simulink model "detumbling1"  (R2022b)
settings: Solver=ode5  StartTime=startTime  StopTime=stopTime  FixedStep=stepsize  RelTol=1e-3
undefined symbols (not defined in the file): a, A_BN0, ARW, c, detumblingkb, detumblingkp, e, EHAccuracy, EHSampleRate, first_detumbling_time_1RW, G, GyroSampleRate, H, h_RW_max, i, inertia1, inertia2, inertia3, Inertia_matrix, Inverse_inertia, Ld, Lw, m, maxdipole, MB, MMnoise, MMSampleRate, mu, n, R_e, rho_d_MB, rho_d_SP, rho_s_MB, rho_s_SP, RRW, SP, theta0, torque_RW_max, w0, wheel_axis
libraries: matrix_library x11, vrlib x10, simulink_extras x4
(part 2 of 3)

== system detumbling1/External Torques/Solar radiation/Torque arm SP ==
  SP : Inport
  A_vect_SP : Inport  Port=2
  S_B : Inport  Port=3
  pointer_SP : Inport  Port=4
  r_SP1 : Inport  Port=5
  r_SP2 : Inport  Port=6
  Add : Sum
  Add1 : Sum
  Reshape : Reshape  OutputDimensionality=Customize  OutputDimensions=[2,3]
  Vector Concatenate : Concatenate
  creazione raggi vettore tra CM SP e centro facce illuminate della faccia che ha come normale l'asse j : Subsystem
  distance : Outport
  wires:
  Reshape/1 -> distance/1
  SP/1 -> [SP]
  A_vect_SP/1 -> [A_vect_SP]
  S_B/1 -> [S_B]
  pointer_SP/1 -> [pointer_SP]
  r_SP1/1 -> [r_SP1]
  r_SP2/1 -> [r_SP2]
  [S_B] -> creazione raggi vettore tra CM SP e centro facce illuminate della faccia che ha come normale l'asse j/1(S_B)
  [SP] -> creazione raggi vettore tra CM SP e centro facce illuminate della faccia che ha come normale l'asse j/2(SP)
  [A_vect_SP] -> creazione raggi vettore tra CM SP e centro facce illuminate della faccia che ha come normale l'asse j/3(A_vect)
  [pointer_SP] -> creazione raggi vettore tra CM SP e centro facce illuminate della faccia che ha come normale l'asse j/4(pointer)
  creazione raggi vettore tra CM SP e centro facce illuminate della faccia che ha come normale l'asse j/1(distance) -> [distance]
  Vector Concatenate/1 -> Reshape/1
  Add/1 -> Vector Concatenate/1
  [distance] -> Add/1
  [r_SP1] -> Add/2
  [r_SP2] -> Add1/2
  [distance] -> Add1/1
  Add1/1 -> Vector Concatenate/2

== system detumbling1/Sensors/Earth Horizon Sensor/A_eps ==
  Constant : Constant
  Display : Display
  Gain : Gain  Gain=[1; -1; 1]
  Gain1 : Gain  Gain=[1; 1; -1]
  Gain2 : Gain  Gain=[-1; 1; 1]
  Matrix Concatenate : Concatenate  NumInputs=3  Mode=Multidimensional array  ConcatenateDimension=2
  Random Number : RandomNumber  Variance=deg2rad(EHAccuracy)^2  Seed=5  SampleTime=1/EHSampleRate
  Random Number1 : RandomNumber  Variance=deg2rad(EHAccuracy)^2  Seed=6  SampleTime=1/EHSampleRate
  Random Number2 : RandomNumber  Variance=deg2rad(EHAccuracy)^2  Seed=7  SampleTime=1/EHSampleRate
  Selector : Selector  InputPortWidth=4  IndexOptions=Index vector (dialog)  Indices=[1 4 3]  OutputSizes=1
  Selector1 : Selector  InputPortWidth=4  IndexOptions=Index vector (dialog)  Indices=[4 1 2 ]  OutputSizes=1
  Selector2 : Selector  InputPortWidth=4  IndexOptions=Index vector (dialog)  Indices=[3 2 1]  OutputSizes=1
  Vector Concatenate : Concatenate  NumInputs=4
  A_epsHS : Outport
  wires:
  Selector/1 -> Gain/1
  Matrix Concatenate/1 -> A_epsHS/1, Display/1
  Random Number/1 -> Vector Concatenate/2
  Vector Concatenate/1 -> Selector2/1, Selector/1, Selector1/1
  Selector1/1 -> Gain1/1
  Gain/1 -> Matrix Concatenate/1
  Selector2/1 -> Gain2/1
  Gain2/1 -> Matrix Concatenate/3
  Gain1/1 -> Matrix Concatenate/2
  Constant/1 -> Vector Concatenate/1
  Random Number2/1 -> Vector Concatenate/4
  Random Number1/1 -> Vector Concatenate/3

== system detumbling1/Sensors/Magnetometer/Subsystem ==
  Constant : Constant
  Display : Display
  Gain : Gain  Gain=[1; -1; 1]
  Gain1 : Gain  Gain=[1; 1; -1]
  Gain2 : Gain  Gain=[-1; 1; 1]
  Matrix Concatenate : Concatenate  NumInputs=3  Mode=Multidimensional array  ConcatenateDimension=2
  Random Number : RandomNumber  Variance=deg2rad(0.1)^2  Seed=5  SampleTime=1/MMSampleRate
  Random Number1 : RandomNumber  Variance=deg2rad(0.1)^2  Seed=6  SampleTime=1/MMSampleRate
  Random Number2 : RandomNumber  Variance=deg2rad(0.1)^2  Seed=7  SampleTime=1/MMSampleRate
  Selector : Selector  InputPortWidth=4  IndexOptions=Index vector (dialog)  Indices=[1 4 3]  OutputSizes=1
  Selector1 : Selector  InputPortWidth=4  IndexOptions=Index vector (dialog)  Indices=[4 1 2]  OutputSizes=1
  Selector2 : Selector  InputPortWidth=4  IndexOptions=Index vector (dialog)  Indices=[3 2 1]  OutputSizes=1
  Vector Concatenate : Concatenate  NumInputs=4
  A_epsMM : Outport
  wires:
  Selector2/1 -> Gain2/1
  Selector/1 -> Gain/1
  Gain/1 -> Matrix Concatenate/1
  Random Number/1 -> Vector Concatenate/2
  Matrix Concatenate/1 -> Display/1, A_epsMM/1
  Selector1/1 -> Gain1/1
  Vector Concatenate/1 -> Selector2/1, Selector/1, Selector1/1
  Gain2/1 -> Matrix Concatenate/3
  Constant/1 -> Vector Concatenate/1
  Gain1/1 -> Matrix Concatenate/2
  Random Number2/1 -> Vector Concatenate/4
  Random Number1/1 -> Vector Concatenate/3

== system detumbling1/External Torques/Solar radiation/Force MB/Subsystem ==
  S_B : Inport
  N_MB : Inport  Port=2
  Constant3 : Constant  Value=[1, 1, 1]
  Matrix Multiply5 : Product  Multiplication=Matrix(*)
  Product10 : Product
  Reshape11 : Reshape  OutputDimensionality=Row vector (2-D)
  Reshape12 : Reshape  OutputDimensionality=Column vector (2-D)
  Sum of Elements : Sum  Inputs=+  CollapseMode=Specified dimension  CollapseDim=2
  Out1 : Outport
  wires:
  Matrix Multiply5/1 -> Product10/1
  Reshape12/1 -> Matrix Multiply5/1
  S_B/1 -> Reshape12/1
  Product10/1 -> Sum of Elements/1
  N_MB/1 -> Product10/2
  Sum of Elements/1 -> Out1/1
  Constant3/1 -> Reshape11/1
  Reshape11/1 -> Matrix Multiply5/2

== system detumbling1/External Torques/Solar radiation/Inertia matrix/r_SP ==
  b_SP : Inport
  a_MB : Inport  Port=2
  Constant : Constant  Value=[1 0 0]
  Gain : Gain  Gain=1/2
  Gain1 : Gain  Gain=1/2
  Gain2 : Gain  Gain=-1
  Product : Product
  Reshape : Reshape  OutputDimensionality=Column vector (2-D)
  Sum : Sum
  r_SP1 : Outport
  r_SP2 : Outport  Port=2
  wires:
  Constant/1 -> Reshape/1
  a_MB/1 -> Gain/1
  b_SP/1 -> Gain1/1
  Gain1/1 -> Sum/1
  Gain/1 -> Sum/2
  Reshape/1 -> Product/1
  Sum/1 -> Product/2
  Gain2/1 -> r_SP2/1
  Product/1 -> r_SP1/1, Gain2/1

== system detumbling1/External Torques/Solar radiation/S_B dot N_MB/If Action Subsystem ==
  NMB : Inport
  Action Port : ActionPort  ActionPortLabel=if(u1 > 0)
  Constant : Constant
  Selector : Selector  NumberOfDimensions=2  InputPortWidth=3  IndexOptions=Index vector (dialog),Index vector (dialog)  Indices=1,[1 2 3]  OutputSizes=1,1
  x : Outport
  pointer : Outport  Port=2
  wires:
  NMB/1 -> Selector/1
  Selector/1 -> x/1
  Constant/1 -> pointer/1

== system detumbling1/External Torques/Solar radiation/S_B dot N_MB/If Action Subsystem1 ==
  NMB : Inport
  Action Port : ActionPort  ActionPortLabel=if(u1 > 0)
  Constant : Constant
  Selector : Selector  NumberOfDimensions=2  InputPortWidth=3  IndexOptions=Index vector (dialog),Index vector (dialog)  Indices=2,[1 2 3]  OutputSizes=1,1
  y : Outport
  pointer : Outport  Port=2
  wires:
  Selector/1 -> y/1
  NMB/1 -> Selector/1
  Constant/1 -> pointer/1

== system detumbling1/External Torques/Solar radiation/S_B dot N_MB/If Action Subsystem2 ==
  NMB : Inport
  Action Port : ActionPort  ActionPortLabel=if(u1 > 0)
  Constant : Constant
  Selector : Selector  NumberOfDimensions=2  InputPortWidth=3  IndexOptions=Index vector (dialog),Index vector (dialog)  Indices=3,[1 2 3]  OutputSizes=1,1
  z : Outport
  pointer : Outport  Port=2
  wires:
  NMB/1 -> Selector/1
  Selector/1 -> z/1
  Constant/1 -> pointer/1

== system detumbling1/External Torques/Solar radiation/S_B dot N_MB/If Action Subsystem3 ==
  NMB : Inport
  Action Port : ActionPort  ActionPortLabel=else
  Constant : Constant  Value=-1
  Selector : Selector  NumberOfDimensions=2  InputPortWidth=3  IndexOptions=Index vector (dialog),Index vector (dialog)  Indices=4,[1 2 3]  OutputSizes=1,1
  -x : Outport
  pointer : Outport  Port=2
  wires:
  Selector/1 -> -x/1
  NMB/1 -> Selector/1
  Constant/1 -> pointer/1

== system detumbling1/External Torques/Solar radiation/S_B dot N_MB/If Action Subsystem4 ==
  NMB : Inport
  Action Port : ActionPort  ActionPortLabel=else
  Constant : Constant  Value=-1
  Selector : Selector  NumberOfDimensions=2  InputPortWidth=3  IndexOptions=Index vector (dialog),Index vector (dialog)  Indices=5,[1 2 3]  OutputSizes=1,1
  -y : Outport
  pointer : Outport  Port=2
  wires:
  NMB/1 -> Selector/1
  Selector/1 -> -y/1
  Constant/1 -> pointer/1

== system detumbling1/External Torques/Solar radiation/S_B dot N_MB/If Action Subsystem5 ==
  NMB : Inport
  Action Port : ActionPort  ActionPortLabel=else
  Constant : Constant  Value=-1
  Selector : Selector  NumberOfDimensions=2  InputPortWidth=3  IndexOptions=Index vector (dialog),Index vector (dialog)  Indices=6,[1 2 3]  OutputSizes=1,1
  -z : Outport
  pointer : Outport  Port=2
  wires:
  Selector/1 -> -z/1
  NMB/1 -> Selector/1
  Constant/1 -> pointer/1

== system detumbling1/External Torques/Solar radiation/S_B dot N_SP/If Action Subsystem ==
  N_SP : Inport
  Action Port : ActionPort  ActionPortLabel=if(u1 > 0)
  Constant : Constant
  Selector : Selector  NumberOfDimensions=2  InputPortWidth=3  IndexOptions=Index vector (dialog),Index vector (dialog)  Indices=1,[1 2 3]  OutputSizes=1,1
  true_NSP : Outport
  pointer : Outport  Port=2
  wires:
  N_SP/1 -> Selector/1
  Constant/1 -> pointer/1
  Selector/1 -> true_NSP/1

== system detumbling1/External Torques/Solar radiation/S_B dot N_SP/If Action Subsystem1 ==
  N_SP : Inport
  Action Port : ActionPort  ActionPortLabel=if(u1 > 0)
  Constant : Constant  Value=-1
  Selector : Selector  NumberOfDimensions=2  InputPortWidth=3  IndexOptions=Index vector (dialog),Index vector (dialog)  Indices=2,[1 2 3]  OutputSizes=1,1
  true_NSP : Outport
  pointer : Outport  Port=2
  wires:
  Selector/1 -> true_NSP/1
  Constant/1 -> pointer/1
  N_SP/1 -> Selector/1

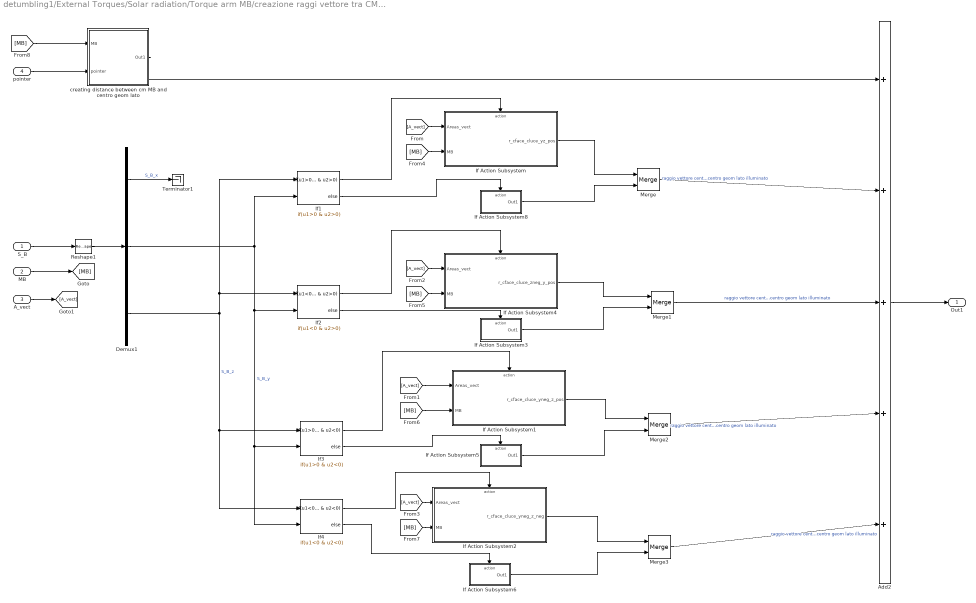
== system detumbling1/External Torques/Solar radiation/Torque arm MB/creazione raggi vettore tra CM MB e centro facce illuminate della faccia che ha come normale l'asse i ==
  S_B : Inport
  MB : Inport  Port=2
  A_vect : Inport  Port=3
  pointer : Inport  Port=4
  Add2 : Sum  Inputs=+|+|+|+|+
  Demux1 : Demux  Outputs=3
  If Action Subsystem : Subsystem  TreatAsAtomicUnit=on
  If Action Subsystem1 : Subsystem  TreatAsAtomicUnit=on
  If Action Subsystem2 : Subsystem  TreatAsAtomicUnit=on
  If Action Subsystem3 : Subsystem  TreatAsAtomicUnit=on
  If Action Subsystem4 : Subsystem  TreatAsAtomicUnit=on
  If Action Subsystem5 : Subsystem  TreatAsAtomicUnit=on
  If Action Subsystem6 : Subsystem  TreatAsAtomicUnit=on
  If Action Subsystem8 : Subsystem  TreatAsAtomicUnit=on
  If1 : If  NumInputs=2  IfExpression=u1>0 & u2>0
  If2 : If  NumInputs=2  IfExpression=u1<0 & u2>0
  If3 : If  NumInputs=2  IfExpression=u1>0 & u2<0
  If4 : If  NumInputs=2  IfExpression=u1<0 & u2<0
  Merge{,1..3} (4 alike) : Merge
  Reshape1 : Reshape  OutputDimensionality=Column vector (2-D)
  Terminator1 : Terminator
  creating distance between cm MB and centro geom lato : Subsystem
  Out1 : Outport
  wires:
  [A_vect] -> If Action Subsystem2/1(Areas_vect)
  [A_vect] -> If Action Subsystem1/1(Areas_vect)
  [A_vect] -> If Action Subsystem4/1(Areas_vect)
  Add2/1 -> Out1/1
  Merge3/1 -> Add2/5  "raggio vettore centro geom lato- centro geom lato illuminato"
  If4/1 -> If Action Subsystem2/Action
  If Action Subsystem2/1(r_cface_cluce_yneg_z_neg) -> Merge3/1
  If3/1 -> If Action Subsystem1/Action
  [A_vect] -> If Action Subsystem/1(Areas_vect)
  Merge1/1 -> Add2/3  "raggio vettore centro geom lato- centro geom lato illuminato"
  If Action Subsystem4/1(r_cface_cluce_zneg_y_pos) -> Merge1/1
  Merge/1 -> Add2/2  "raggio vettore centro geom lato- centro geom lato illuminato"
  If Action Subsystem/1(r_cface_cluce_yz_pos) -> Merge/1
  If1/2 -> If Action Subsystem8/Action
  S_B/1 -> Reshape1/1
  Reshape1/1 -> Demux1/1
  Demux1/2 -> If2/2, If3/2, If4/2, If1/2  "S_B_y"
  If2/1 -> If Action Subsystem4/Action
  If1/1 -> If Action Subsystem/Action
  Demux1/3 -> If4/1, If3/1, If2/1, If1/1  "S_B_z"
  creating distance between cm MB and centro geom lato/1(Out1) -> Add2/1
  Demux1/1 -> Terminator1/1  "S_B_x"
  MB/1 -> [MB]
  [MB] -> If Action Subsystem/2(MB)
  [MB] -> If Action Subsystem4/2(MB)
  [MB] -> If Action Subsystem1/2(MB)
  [MB] -> If Action Subsystem2/2(MB)
  If Action Subsystem8/1(Out1) -> Merge/2
  If2/2 -> If Action Subsystem3/Action
  If3/2 -> If Action Subsystem5/Action
  If4/2 -> If Action Subsystem6/Action
  If Action Subsystem3/1(Out1) -> Merge1/2
  If Action Subsystem1/1(r_cface_cluce_yneg_z_pos) -> Merge2/1
  If Action Subsystem5/1(Out1) -> Merge2/2
  Merge2/1 -> Add2/4  "raggio vettore centro geom lato- centro geom lato illuminato"
  If Action Subsystem6/1(Out1) -> Merge3/2
  [MB] -> creating distance between cm MB and centro geom lato/1(MB)
  A_vect/1 -> [A_vect]
  pointer/1 -> creating distance between cm MB and centro geom lato/2(pointer)

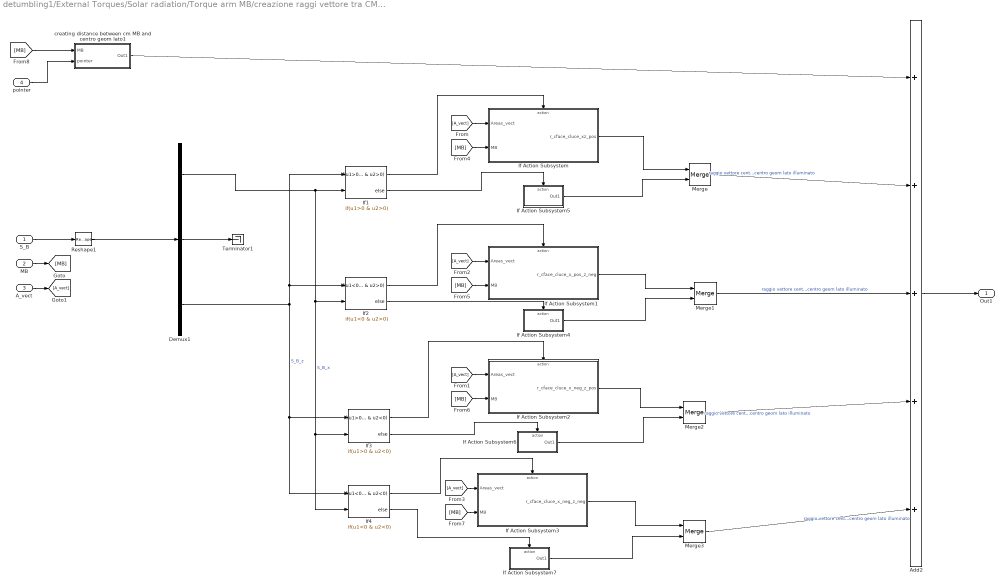
== system detumbling1/External Torques/Solar radiation/Torque arm MB/creazione raggi vettore tra CM MB e centro facce illuminate della faccia che ha come normale l'asse j ==
  S_B : Inport
  MB : Inport  Port=2
  A_vect : Inport  Port=3
  pointer : Inport  Port=4
  Add2 : Sum  Inputs=+|+|+|+|+
  Demux1 : Demux  Outputs=3
  If Action Subsystem : Subsystem  TreatAsAtomicUnit=on
  If Action Subsystem1 : Subsystem  TreatAsAtomicUnit=on
  If Action Subsystem2 : Subsystem  TreatAsAtomicUnit=on
  If Action Subsystem3 : Subsystem  TreatAsAtomicUnit=on
  If Action Subsystem4 : Subsystem  TreatAsAtomicUnit=on
  If Action Subsystem5 : Subsystem  TreatAsAtomicUnit=on
  If Action Subsystem6 : Subsystem  TreatAsAtomicUnit=on
  If Action Subsystem7 : Subsystem  TreatAsAtomicUnit=on
  If1 : If  NumInputs=2  IfExpression=u1>0 & u2>0
  If2 : If  NumInputs=2  IfExpression=u1<0 & u2>0
  If3 : If  NumInputs=2  IfExpression=u1>0 & u2<0
  If4 : If  NumInputs=2  IfExpression=u1<0 & u2<0
  Merge{,1..3} (4 alike) : Merge
  Reshape1 : Reshape  OutputDimensionality=Column vector (2-D)
  Terminator1 : Terminator
  creating distance between cm MB and centro geom lato1 : Subsystem
  Out1 : Outport
  wires:
  Demux1/2 -> Terminator1/1
  creating distance between cm MB and centro geom lato1/1(Out1) -> Add2/1
  If1/1 -> If Action Subsystem/Action
  If2/1 -> If Action Subsystem1/Action
  Reshape1/1 -> Demux1/1
  S_B/1 -> Reshape1/1
  If Action Subsystem/1(r_cface_cluce_xz_pos) -> Merge/1
  Merge/1 -> Add2/2  "raggio vettore centro geom lato- centro geom lato illuminato"
  If Action Subsystem1/1(r_cface_cluce_x_pos_z_neg) -> Merge1/1
  Merge1/1 -> Add2/3  "raggio vettore centro geom lato- centro geom lato illuminato"
  [A_vect] -> If Action Subsystem/1(Areas_vect)
  Merge2/1 -> Add2/4  "raggio vettore centro geom lato- centro geom lato illuminato"
  If3/1 -> If Action Subsystem2/Action
  If Action Subsystem3/1(r_cface_cluce_x_neg_z_neg) -> Merge3/1
  If4/1 -> If Action Subsystem3/Action
  Merge3/1 -> Add2/5  "raggio vettore centro geom lato- centro geom lato illuminato"
  Add2/1 -> Out1/1
  [A_vect] -> If Action Subsystem1/1(Areas_vect)
  [A_vect] -> If Action Subsystem2/1(Areas_vect)
  [A_vect] -> If Action Subsystem3/1(Areas_vect)
  Demux1/3 -> If4/1, If3/1, If2/1, If1/1  "S_B_z"
  Demux1/1 -> If1/2, If4/2, If3/2, If2/2  "S_B_x"
  MB/1 -> [MB]
  [MB] -> If Action Subsystem/2(MB)
  [MB] -> If Action Subsystem1/2(MB)
  [MB] -> If Action Subsystem2/2(MB)
  [MB] -> If Action Subsystem3/2(MB)
  If1/2 -> If Action Subsystem5/Action
  If2/2 -> If Action Subsystem4/Action
  If3/2 -> If Action Subsystem6/Action
  If4/2 -> If Action Subsystem7/Action
  If Action Subsystem5/1(Out1) -> Merge/2
  If Action Subsystem4/1(Out1) -> Merge1/2
  If Action Subsystem2/1(r_cface_cluce_x_neg_z_pos) -> Merge2/1
  If Action Subsystem6/1(Out1) -> Merge2/2
  If Action Subsystem7/1(Out1) -> Merge3/2
  [MB] -> creating distance between cm MB and centro geom lato1/1(MB)
  A_vect/1 -> [A_vect]
  pointer/1 -> creating distance between cm MB and centro geom lato1/2(pointer)

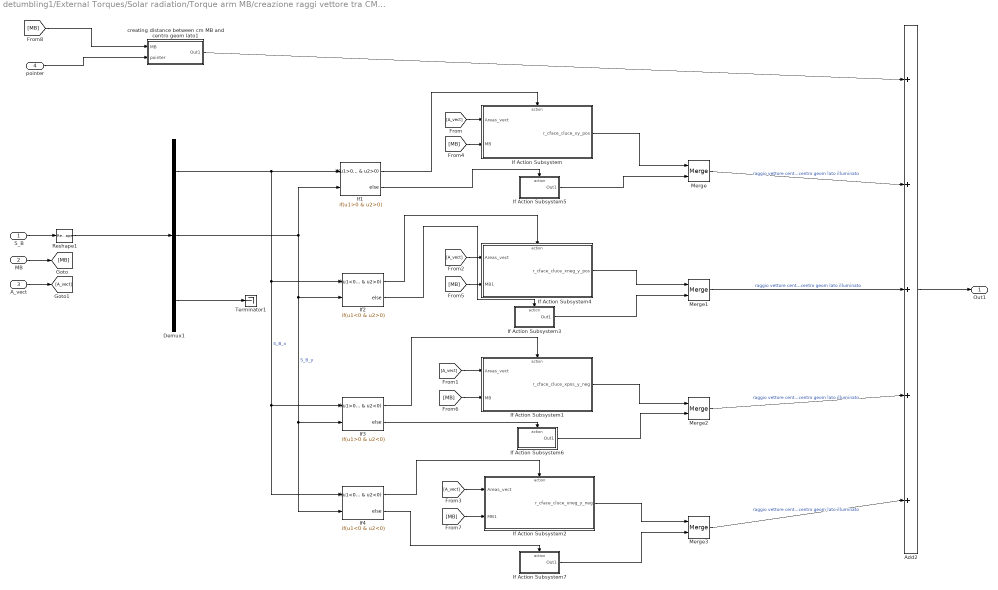
== system detumbling1/External Torques/Solar radiation/Torque arm MB/creazione raggi vettore tra CM MB e centro facce illuminate della faccia che ha come normale l'asse k ==
  S_B : Inport
  MB : Inport  Port=2
  A_vect : Inport  Port=3
  pointer : Inport  Port=4
  Add2 : Sum  Inputs=+|+|+|+|+
  Demux1 : Demux  Outputs=3
  If Action Subsystem : Subsystem  TreatAsAtomicUnit=on
  If Action Subsystem1 : Subsystem  TreatAsAtomicUnit=on
  If Action Subsystem2 : Subsystem  TreatAsAtomicUnit=on
  If Action Subsystem3 : Subsystem  TreatAsAtomicUnit=on
  If Action Subsystem4 : Subsystem  TreatAsAtomicUnit=on
  If Action Subsystem5 : Subsystem  TreatAsAtomicUnit=on
  If Action Subsystem6 : Subsystem  TreatAsAtomicUnit=on
  If Action Subsystem7 : Subsystem  TreatAsAtomicUnit=on
  If1 : If  NumInputs=2  IfExpression=u1>0 & u2>0
  If2 : If  NumInputs=2  IfExpression=u1<0 & u2>0
  If3 : If  NumInputs=2  IfExpression=u1>0 & u2<0
  If4 : If  NumInputs=2  IfExpression=u1<0 & u2<0
  Merge{,1..3} (4 alike) : Merge
  Reshape1 : Reshape  OutputDimensionality=Column vector (2-D)
  Terminator1 : Terminator
  creating distance between cm MB and centro geom lato1 : Subsystem
  Out1 : Outport
  wires:
  Demux1/3 -> Terminator1/1
  Demux1/1 -> If1/1, If4/1, If3/1, If2/1  "S_B_x"
  If1/1 -> If Action Subsystem/Action
  If2/1 -> If Action Subsystem4/Action
  Demux1/2 -> If4/2, If3/2, If2/2, If1/2  "S_B_y"
  Reshape1/1 -> Demux1/1
  S_B/1 -> Reshape1/1
  If1/2 -> If Action Subsystem5/Action
  Merge/1 -> Add2/2  "raggio vettore centro geom lato- centro geom lato illuminato"
  Merge1/1 -> Add2/3  "raggio vettore centro geom lato- centro geom lato illuminato"
  [A_vect] -> If Action Subsystem/1(Areas_vect)
  Merge2/1 -> Add2/4  "raggio vettore centro geom lato- centro geom lato illuminato"
  If3/2 -> If Action Subsystem6/Action
  If Action Subsystem1/1(r_cface_cluce_xpos_y_neg) -> Merge2/1
  If3/1 -> If Action Subsystem1/Action
  If4/2 -> If Action Subsystem7/Action
  If4/1 -> If Action Subsystem2/Action
  Merge3/1 -> Add2/5  "raggio vettore centro geom lato- centro geom lato illuminato"
  Add2/1 -> Out1/1
  [A_vect] -> If Action Subsystem4/1(Areas_vect)
  [A_vect] -> If Action Subsystem1/1(Areas_vect)
  [A_vect] -> If Action Subsystem2/1(Areas_vect)
  MB/1 -> [MB]
  [MB] -> If Action Subsystem/2(MB)
  [MB] -> If Action Subsystem4/2(MB1)
  [MB] -> If Action Subsystem1/2(MB)
  [MB] -> If Action Subsystem2/2(MB1)
  If2/2 -> If Action Subsystem3/Action
  If Action Subsystem/1(r_cface_cluce_xy_pos) -> Merge/1
  If Action Subsystem5/1(Out1) -> Merge/2
  If Action Subsystem4/1(r_cface_cluce_xneg_y_pos) -> Merge1/1
  If Action Subsystem3/1(Out1) -> Merge1/2
  If Action Subsystem6/1(Out1) -> Merge2/2
  If Action Subsystem2/1(r_cface_cluce_xneg_y_neg) -> Merge3/1
  If Action Subsystem7/1(Out1) -> Merge3/2
  [MB] -> creating distance between cm MB and centro geom lato1/1(MB)
  creating distance between cm MB and centro geom lato1/1(Out1) -> Add2/1
  A_vect/1 -> [A_vect]
  pointer/1 -> creating distance between cm MB and centro geom lato1/2(pointer)

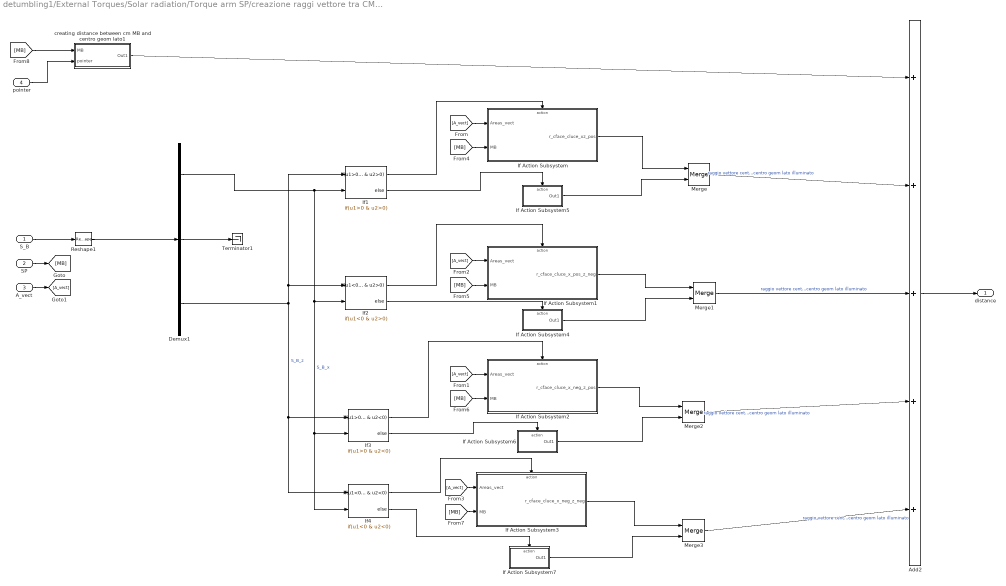
== system detumbling1/External Torques/Solar radiation/Torque arm SP/creazione raggi vettore tra CM SP e centro facce illuminate della faccia che ha come normale l'asse j ==
  S_B : Inport
  SP : Inport  Port=2
  A_vect : Inport  Port=3
  pointer : Inport  Port=4
  Add2 : Sum  Inputs=+|+|+|+|+
  Demux1 : Demux  Outputs=3
  If Action Subsystem : Subsystem  TreatAsAtomicUnit=on
  If Action Subsystem1 : Subsystem  TreatAsAtomicUnit=on
  If Action Subsystem2 : Subsystem  TreatAsAtomicUnit=on
  If Action Subsystem3 : Subsystem  TreatAsAtomicUnit=on
  If Action Subsystem4 : Subsystem  TreatAsAtomicUnit=on
  If Action Subsystem5 : Subsystem  TreatAsAtomicUnit=on
  If Action Subsystem6 : Subsystem  TreatAsAtomicUnit=on
  If Action Subsystem7 : Subsystem  TreatAsAtomicUnit=on
  If1 : If  NumInputs=2  IfExpression=u1>0 & u2>0
  If2 : If  NumInputs=2  IfExpression=u1<0 & u2>0
  If3 : If  NumInputs=2  IfExpression=u1>0 & u2<0
  If4 : If  NumInputs=2  IfExpression=u1<0 & u2<0
  Merge{,1..3} (4 alike) : Merge
  Reshape1 : Reshape  OutputDimensionality=Column vector (2-D)
  Terminator1 : Terminator
  creating distance between cm MB and centro geom lato1 : Subsystem
  distance : Outport
  wires:
  Demux1/2 -> Terminator1/1
  creating distance between cm MB and centro geom lato1/1(Out1) -> Add2/1
  If1/1 -> If Action Subsystem/Action
  If2/1 -> If Action Subsystem1/Action
  Reshape1/1 -> Demux1/1
  S_B/1 -> Reshape1/1
  If Action Subsystem/1(r_cface_cluce_xz_pos) -> Merge/1
  Merge/1 -> Add2/2  "raggio vettore centro geom lato- centro geom lato illuminato"
  If Action Subsystem1/1(r_cface_cluce_x_pos_z_neg) -> Merge1/1
  Merge1/1 -> Add2/3  "raggio vettore centro geom lato- centro geom lato illuminato"
  [A_vect] -> If Action Subsystem/1(Areas_vect)
  Merge2/1 -> Add2/4  "raggio vettore centro geom lato- centro geom lato illuminato"
  If3/1 -> If Action Subsystem2/Action
  If Action Subsystem3/1(r_cface_cluce_x_neg_z_neg) -> Merge3/1
  If4/1 -> If Action Subsystem3/Action
  Merge3/1 -> Add2/5  "raggio vettore centro geom lato- centro geom lato illuminato"
  Add2/1 -> distance/1
  [A_vect] -> If Action Subsystem1/1(Areas_vect)
  [A_vect] -> If Action Subsystem2/1(Areas_vect)
  [A_vect] -> If Action Subsystem3/1(Areas_vect)
  Demux1/3 -> If4/1, If3/1, If2/1, If1/1  "S_B_z"
  Demux1/1 -> If1/2, If4/2, If3/2, If2/2  "S_B_x"
  SP/1 -> [MB]
  [MB] -> If Action Subsystem/2(MB)
  [MB] -> If Action Subsystem1/2(MB)
  [MB] -> If Action Subsystem2/2(MB)
  [MB] -> If Action Subsystem3/2(MB)
  If1/2 -> If Action Subsystem5/Action
  If2/2 -> If Action Subsystem4/Action
  If3/2 -> If Action Subsystem6/Action
  If4/2 -> If Action Subsystem7/Action
  If Action Subsystem5/1(Out1) -> Merge/2
  If Action Subsystem4/1(Out1) -> Merge1/2
  If Action Subsystem2/1(r_cface_cluce_x_neg_z_pos) -> Merge2/1
  If Action Subsystem6/1(Out1) -> Merge2/2
  If Action Subsystem7/1(Out1) -> Merge3/2
  [MB] -> creating distance between cm MB and centro geom lato1/1(MB)
  A_vect/1 -> [A_vect]
  pointer/1 -> creating distance between cm MB and centro geom lato1/2(pointer)

== system detumbling1/External Torques/Solar radiation/Torque arm MB/creazione raggi vettore tra CM MB e centro facce illuminate della faccia che ha come normale l'asse i/If Action Subsystem ==
  Areas_vect : Inport
  MB : Inport  Port=2
  Action Port : ActionPort  ActionPortLabel=if(u1>0 & u2>0)
  Add : Sum  Inputs=+|-
  Add1 : Sum  Inputs=+|-
  Add2 : Sum
  Demux : Demux  Outputs=3
  Demux2 : Demux
  Divide : Product  Inputs=*/
  Divide1 : Product  Inputs=*/
  Gain{,1..3} (4 alike) : Gain  Gain=1/2
  Ground : Ground
  Ground1 : Ground
  Mux : Mux  Inputs=3
  Mux1 : Mux  Inputs=3
  Reshape : Reshape  OutputDimensionality=Column vector (2-D)
  Reshape2 : Reshape  OutputDimensionality=Column vector (2-D)
  Reshape3 : Reshape  OutputDimensionality=Column vector (2-D)
  Terminator{1..2,8..9} (4 alike) : Terminator
  r_cface_cluce_yz_pos : Outport
  wires:
  Demux/2 -> Terminator8/1
  Demux/3 -> Terminator9/1
  Add2/1 -> r_cface_cluce_yz_pos/1
  Reshape3/1 -> Add2/2
  Reshape2/1 -> Add2/1
  [h_MB] -> Gain2/1
  Divide1/1 -> Gain3/1
  Gain2/1 -> Add1/1
  Gain3/1 -> Add1/2
  Ground/1 -> Mux1/2, Mux1/1
  Mux1/1 -> Reshape3/1  "raggio vettore che collega il centro geom della faccia con il centro geom della faccia illuminata dal sole lungo k"
  [b_MB] -> Divide1/2
  Reshape/1 -> Demux/1
  Ground1/1 -> Mux/3, Mux/1
  Areas_vect/1 -> Reshape/1
  [h_MB] -> Divide/2
  Gain/1 -> Add/1
  [b_MB] -> Gain/1
  Gain1/1 -> Add/2
  Mux/1 -> Reshape2/1  "raggio vettore che collega il centro geom della faccia con il centro geom della faccia illuminata dal sole lungo j"
  Divide/1 -> Gain1/1
  Demux/1 -> Divide1/1, Divide/1
  Add/1 -> Mux/2
  Add1/1 -> Mux1/3
  Demux2/1 -> Terminator2/1
  Demux2/2 -> Terminator1/1
  MB/1 -> Demux2/1
  Demux2/3 -> [b_MB]
  Demux2/4 -> [h_MB]

== system detumbling1/External Torques/Solar radiation/Torque arm MB/creazione raggi vettore tra CM MB e centro facce illuminate della faccia che ha come normale l'asse i/If Action Subsystem1 ==
  Areas_vect : Inport
  MB : Inport  Port=2
  Action Port : ActionPort  ActionPortLabel=if(u1>0 & u2<0)
  Add : Sum  Inputs=+|-
  Add1 : Sum  Inputs=+|-
  Add2 : Sum
  Demux : Demux  Outputs=3
  Demux2 : Demux
  Divide : Product  Inputs=*/
  Divide1 : Product  Inputs=*/
  Gain{,1..3} (4 alike) : Gain  Gain=1/2
  Gain4 : Gain  Gain=-1
  Ground : Ground
  Ground1 : Ground
  Mux : Mux  Inputs=3
  Mux1 : Mux  Inputs=3
  Reshape : Reshape  OutputDimensionality=Column vector (2-D)
  Reshape2 : Reshape  OutputDimensionality=Column vector (2-D)
  Reshape3 : Reshape  OutputDimensionality=Column vector (2-D)
  Terminator{1..2,8..9} (4 alike) : Terminator
  r_cface_cluce_yneg_z_pos : Outport
  wires:
  Add1/1 -> Mux1/3
  Demux/1 -> Divide/1, Divide1/1
  Divide/1 -> Gain1/1
  Mux/1 -> Reshape2/1  "raggio vettore che collega il centro geom della faccia con il centro geom della faccia illuminata dal sole lungo -j"
  Gain1/1 -> Add/2
  [b_MB] -> Gain/1
  Gain/1 -> Add/1
  [h_MB] -> Divide/2
  Areas_vect/1 -> Reshape/1
  Ground1/1 -> Mux/1, Mux/3
  Reshape/1 -> Demux/1
  [b_MB] -> Divide1/2
  Mux1/1 -> Reshape3/1  "raggio vettore che collega il centro geom della faccia con il centro geom della faccia illuminata dal sole lungo k"
  Ground/1 -> Mux1/1, Mux1/2
  Gain3/1 -> Add1/2
  Gain2/1 -> Add1/1
  Divide1/1 -> Gain3/1
  [h_MB] -> Gain2/1
  Reshape2/1 -> Add2/1
  Reshape3/1 -> Add2/2
  Add2/1 -> r_cface_cluce_yneg_z_pos/1
  Demux/3 -> Terminator9/1
  Demux/2 -> Terminator8/1
  Add/1 -> Gain4/1
  Gain4/1 -> Mux/2
  Demux2/1 -> Terminator2/1
  Demux2/2 -> Terminator1/1
  MB/1 -> Demux2/1
  Demux2/3 -> [b_MB]
  Demux2/4 -> [h_MB]

== system detumbling1/External Torques/Solar radiation/Torque arm MB/creazione raggi vettore tra CM MB e centro facce illuminate della faccia che ha come normale l'asse i/If Action Subsystem2 ==
  Areas_vect : Inport
  MB : Inport  Port=2
  Action Port : ActionPort  ActionPortLabel=if(u1<0 & u2<0)
  Add : Sum  Inputs=+|-
  Add1 : Sum  Inputs=+|-
  Add2 : Sum
  Demux : Demux  Outputs=3
  Demux2 : Demux
  Divide : Product  Inputs=*/
  Divide1 : Product  Inputs=*/
  Gain{,1..3} (4 alike) : Gain  Gain=1/2
  Gain4 : Gain  Gain=-1
  Gain5 : Gain  Gain=-1
  Ground : Ground
  Ground1 : Ground
  Mux : Mux  Inputs=3
  Mux1 : Mux  Inputs=3
  Reshape : Reshape  OutputDimensionality=Column vector (2-D)
  Reshape2 : Reshape  OutputDimensionality=Column vector (2-D)
  Reshape3 : Reshape  OutputDimensionality=Column vector (2-D)
  Terminator{1..2,8..9} (4 alike) : Terminator
  r_cface_cluce_yneg_z_neg : Outport
  wires:
  Gain4/1 -> Mux/2
  Add/1 -> Gain4/1
  Demux/2 -> Terminator8/1
  Demux/3 -> Terminator9/1
  Add2/1 -> r_cface_cluce_yneg_z_neg/1
  Reshape3/1 -> Add2/2
  Reshape2/1 -> Add2/1
  [h_MB] -> Gain2/1
  Divide1/1 -> Gain3/1
  Gain2/1 -> Add1/1
  Gain3/1 -> Add1/2
  Ground/1 -> Mux1/2, Mux1/1
  Mux1/1 -> Reshape3/1  "raggio vettore che collega il centro geom della faccia con il centro geom della faccia illuminata dal sole lungo -k"
  [b_MB] -> Divide1/2
  Reshape/1 -> Demux/1
  Ground1/1 -> Mux/3, Mux/1
  Areas_vect/1 -> Reshape/1
  [h_MB] -> Divide/2
  Gain/1 -> Add/1
  [b_MB] -> Gain/1
  Gain1/1 -> Add/2
  Mux/1 -> Reshape2/1  "raggio vettore che collega il centro geom della faccia con il centro geom della faccia illuminata dal sole lungo -j"
  Divide/1 -> Gain1/1
  Demux/1 -> Divide1/1, Divide/1
  Gain5/1 -> Mux1/3
  Add1/1 -> Gain5/1
  Demux2/1 -> Terminator2/1
  Demux2/2 -> Terminator1/1
  MB/1 -> Demux2/1
  Demux2/3 -> [b_MB]
  Demux2/4 -> [h_MB]

== system detumbling1/External Torques/Solar radiation/Torque arm MB/creazione raggi vettore tra CM MB e centro facce illuminate della faccia che ha come normale l'asse i/If Action Subsystem3 ==
  Action Port : ActionPort  ActionPortLabel=else
  Constant : Constant  Value=[0;0;0]
  Out1 : Outport
  wires:
  Constant/1 -> Out1/1

== system detumbling1/External Torques/Solar radiation/Torque arm MB/creazione raggi vettore tra CM MB e centro facce illuminate della faccia che ha come normale l'asse i/If Action Subsystem4 ==
  Areas_vect : Inport
  MB : Inport  Port=2
  Action Port : ActionPort  ActionPortLabel=if(u1<0 & u2>0)
  Add : Sum  Inputs=+|-
  Add1 : Sum  Inputs=+|-
  Add2 : Sum
  Demux : Demux  Outputs=3
  Demux2 : Demux
  Divide : Product  Inputs=*/
  Divide1 : Product  Inputs=*/
  Gain{,1..3} (4 alike) : Gain  Gain=1/2
  Gain4 : Gain  Gain=-1
  Ground : Ground
  Ground1 : Ground
  Mux : Mux  Inputs=3
  Mux1 : Mux  Inputs=3
  Reshape : Reshape  OutputDimensionality=Column vector (2-D)
  Reshape2 : Reshape  OutputDimensionality=Column vector (2-D)
  Reshape3 : Reshape  OutputDimensionality=Column vector (2-D)
  Terminator{1..2,8..9} (4 alike) : Terminator
  r_cface_cluce_zneg_y_pos : Outport
  wires:
  [h_MB] -> Divide1/2
  [b_MB] -> Gain2/1
  Add1/1 -> Mux1/2
  Gain4/1 -> Mux/3
  Add/1 -> Gain4/1
  [h_MB] -> Gain/1
  [b_MB] -> Divide/2
  Divide/1 -> Gain1/1
  Mux/1 -> Reshape2/1  "raggio vettore che collega il centro geom della faccia con il centro geom della faccia illuminata dal sole lungo -k"
  Gain1/1 -> Add/2
  Gain/1 -> Add/1
  Areas_vect/1 -> Reshape/1
  Ground1/1 -> Mux/1, Mux/2
  Reshape/1 -> Demux/1
  Mux1/1 -> Reshape3/1  "raggio vettore che collega il centro geom della faccia con il centro geom della faccia illuminata dal sole lungo j"
  Ground/1 -> Mux1/3, Mux1/1
  Gain3/1 -> Add1/2
  Gain2/1 -> Add1/1
  Divide1/1 -> Gain3/1
  Reshape2/1 -> Add2/1
  Reshape3/1 -> Add2/2
  Add2/1 -> r_cface_cluce_zneg_y_pos/1
  Demux/2 -> Terminator9/1
  Demux/3 -> Terminator8/1
  Demux/1 -> Divide1/1, Divide/1
  Demux2/1 -> Terminator2/1
  Demux2/2 -> Terminator1/1
  MB/1 -> Demux2/1
  Demux2/3 -> [b_MB]
  Demux2/4 -> [h_MB]

== system detumbling1/External Torques/Solar radiation/Torque arm MB/creazione raggi vettore tra CM MB e centro facce illuminate della faccia che ha come normale l'asse i/If Action Subsystem5 ==
  Action Port : ActionPort  ActionPortLabel=else
  Constant : Constant  Value=[0;0;0]
  Out1 : Outport
  wires:
  Constant/1 -> Out1/1

== system detumbling1/External Torques/Solar radiation/Torque arm MB/creazione raggi vettore tra CM MB e centro facce illuminate della faccia che ha come normale l'asse i/If Action Subsystem6 ==
  Action Port : ActionPort  ActionPortLabel=else
  Constant : Constant  Value=[0;0;0]
  Out1 : Outport
  wires:
  Constant/1 -> Out1/1

== system detumbling1/External Torques/Solar radiation/Torque arm MB/creazione raggi vettore tra CM MB e centro facce illuminate della faccia che ha come normale l'asse i/If Action Subsystem8 ==
  Action Port : ActionPort  ActionPortLabel=else
  Constant : Constant  Value=[0;0;0]
  Out1 : Outport
  wires:
  Constant/1 -> Out1/1

== system detumbling1/External Torques/Solar radiation/Torque arm MB/creazione raggi vettore tra CM MB e centro facce illuminate della faccia che ha come normale l'asse i/creating distance between cm MB and centro geom lato ==
  MB : Inport
  pointer : Inport  Port=2
  Demux : Demux
  Ground : Ground
  Mux : Mux  Inputs=3
  Product : Product
  Reshape : Reshape  OutputDimensionality=Column vector (2-D)
  Terminator : Terminator
  Terminator1 : Terminator
  Terminator3 : Terminator
  Out1 : Outport
  wires:
  Reshape/1 -> Out1/1
  Mux/1 -> Reshape/1
  MB/1 -> Demux/1
  Demux/1 -> Terminator/1
  Demux/2 -> Terminator1/1
  Ground/1 -> Mux/3, Mux/1
  Demux/4 -> Terminator3/1
  Demux/3 -> Product/1
  Product/1 -> Mux/2
  pointer/1 -> Product/2

== system detumbling1/External Torques/Solar radiation/Torque arm MB/creazione raggi vettore tra CM MB e centro facce illuminate della faccia che ha come normale l'asse j/If Action Subsystem ==
  Areas_vect : Inport
  MB : Inport  Port=2
  Action Port : ActionPort  ActionPortLabel=if(u1>0 & u2>0)
  Add : Sum  Inputs=+|-
  Add1 : Sum  Inputs=+|-
  Add2 : Sum
  Demux : Demux  Outputs=3
  Demux2 : Demux
  Divide : Product  Inputs=*/
  Divide1 : Product  Inputs=*/
  Gain{,1..3} (4 alike) : Gain  Gain=1/2
  Ground : Ground
  Ground1 : Ground
  Mux : Mux  Inputs=3
  Mux1 : Mux  Inputs=3
  Reshape : Reshape  OutputDimensionality=Column vector (2-D)
  Reshape2 : Reshape  OutputDimensionality=Column vector (2-D)
  Reshape3 : Reshape  OutputDimensionality=Column vector (2-D)
  Terminator{1..2,8..9} (4 alike) : Terminator
  r_cface_cluce_xz_pos : Outport
  wires:
  Add/1 -> Mux/3
  Divide/1 -> Gain1/1
  Mux/1 -> Reshape2/1  "raggio vettore che collega il centro geom della faccia con il centro geom della faccia illuminata dal sole lungo k"
  Gain1/1 -> Add/2
  Demux/2 -> Divide1/1, Divide/1
  [h_MB] -> Gain/1
  Gain/1 -> Add/1
  [a_MB] -> Divide/2
  Areas_vect/1 -> Reshape/1
  Ground1/1 -> Mux/2, Mux/1
  Reshape/1 -> Demux/1
  Add1/1 -> Mux1/1
  [h_MB] -> Divide1/2
  Mux1/1 -> Reshape3/1  "raggio vettore che collega il centro geom della faccia con il centro geom della faccia illuminata dal sole lungo i"
  Ground/1 -> Mux1/2, Mux1/3
  Gain3/1 -> Add1/2
  Gain2/1 -> Add1/1
  Divide1/1 -> Gain3/1
  [a_MB] -> Gain2/1
  Reshape2/1 -> Add2/1
  Reshape3/1 -> Add2/2
  Add2/1 -> r_cface_cluce_xz_pos/1
  Demux/1 -> Terminator9/1
  Demux/3 -> Terminator8/1
  Demux2/1 -> Terminator2/1
  Demux2/2 -> [a_MB]
  MB/1 -> Demux2/1
  Demux2/3 -> Terminator1/1
  Demux2/4 -> [h_MB]

== system detumbling1/External Torques/Solar radiation/Torque arm MB/creazione raggi vettore tra CM MB e centro facce illuminate della faccia che ha come normale l'asse j/If Action Subsystem1 ==
  Areas_vect : Inport
  MB : Inport  Port=2
  Action Port : ActionPort  ActionPortLabel=if(u1<0 & u2>0)
  Add : Sum  Inputs=+|-
  Add1 : Sum  Inputs=+|-
  Add2 : Sum
  Demux : Demux  Outputs=3
  Demux2 : Demux
  Divide : Product  Inputs=*/
  Divide1 : Product  Inputs=*/
  Gain{,1..3} (4 alike) : Gain  Gain=1/2
  Gain4 : Gain  Gain=-1
  Ground : Ground
  Ground1 : Ground
  Mux : Mux  Inputs=3
  Mux1 : Mux  Inputs=3
  Reshape : Reshape  OutputDimensionality=Column vector (2-D)
  Reshape2 : Reshape  OutputDimensionality=Column vector (2-D)
  Reshape3 : Reshape  OutputDimensionality=Column vector (2-D)
  Terminator{1..2,8..9} (4 alike) : Terminator
  r_cface_cluce_x_pos_z_neg : Outport
  wires:
  Demux/3 -> Terminator8/1
  Demux/1 -> Terminator9/1
  Add2/1 -> r_cface_cluce_x_pos_z_neg/1
  Reshape3/1 -> Add2/2
  Reshape2/1 -> Add2/1
  [a_MB] -> Gain2/1
  Divide1/1 -> Gain3/1
  Gain2/1 -> Add1/1
  Gain3/1 -> Add1/2
  Ground/1 -> Mux1/3, Mux1/2
  Mux1/1 -> Reshape3/1  "raggio vettore che collega il centro geom della faccia con il centro geom della faccia illuminata dal sole lungo i"
  [h_MB] -> Divide1/2
  Add1/1 -> Mux1/1
  Reshape/1 -> Demux/1
  Ground1/1 -> Mux/1, Mux/2
  Areas_vect/1 -> Reshape/1
  [a_MB] -> Divide/2
  Gain/1 -> Add/1
  [h_MB] -> Gain/1
  Demux/2 -> Divide/1, Divide1/1
  Gain1/1 -> Add/2
  Mux/1 -> Reshape2/1  "raggio vettore che collega il centro geom della faccia con il centro geom della faccia illuminata dal sole lungo -k"
  Divide/1 -> Gain1/1
  Add/1 -> Gain4/1
  Gain4/1 -> Mux/3
  Demux2/1 -> Terminator2/1
  Demux2/2 -> [a_MB]
  MB/1 -> Demux2/1
  Demux2/3 -> Terminator1/1
  Demux2/4 -> [h_MB]

== system detumbling1/External Torques/Solar radiation/Torque arm MB/creazione raggi vettore tra CM MB e centro facce illuminate della faccia che ha come normale l'asse j/If Action Subsystem2 ==
  Areas_vect : Inport
  MB : Inport  Port=2
  Action Port : ActionPort  ActionPortLabel=if(u1>0 & u2<0)
  Add : Sum  Inputs=+|-
  Add1 : Sum  Inputs=+|-
  Add2 : Sum
  Demux : Demux  Outputs=3
  Demux2 : Demux
  Divide : Product  Inputs=*/
  Divide1 : Product  Inputs=*/
  Gain{,1..3} (4 alike) : Gain  Gain=1/2
  Gain4 : Gain  Gain=-1
  Ground : Ground
  Ground1 : Ground
  Mux : Mux  Inputs=3
  Mux1 : Mux  Inputs=3
  Reshape : Reshape  OutputDimensionality=Column vector (2-D)
  Reshape2 : Reshape  OutputDimensionality=Column vector (2-D)
  Reshape3 : Reshape  OutputDimensionality=Column vector (2-D)
  Terminator{1..2,8..9} (4 alike) : Terminator
  r_cface_cluce_x_neg_z_pos : Outport
  wires:
  Add/1 -> Mux/3
  Divide/1 -> Gain1/1
  Mux/1 -> Reshape2/1  "raggio vettore che collega il centro geom della faccia con il centro geom della faccia illuminata dal sole lungo k"
  Gain1/1 -> Add/2
  Demux/2 -> Divide1/1, Divide/1
  [h_MB] -> Gain/1
  Gain/1 -> Add/1
  [a_MB] -> Divide/2
  Areas_vect/1 -> Reshape/1
  Ground1/1 -> Mux/2, Mux/1
  Reshape/1 -> Demux/1
  [h_MB] -> Divide1/2
  Mux1/1 -> Reshape3/1  "raggio vettore che collega il centro geom della faccia con il centro geom della faccia illuminata dal sole lungo -i"
  Ground/1 -> Mux1/2, Mux1/3
  Gain3/1 -> Add1/2
  Gain2/1 -> Add1/1
  Divide1/1 -> Gain3/1
  [a_MB] -> Gain2/1
  Reshape2/1 -> Add2/1
  Reshape3/1 -> Add2/2
  Add2/1 -> r_cface_cluce_x_neg_z_pos/1
  Demux/1 -> Terminator9/1
  Demux/3 -> Terminator8/1
  Gain4/1 -> Mux1/1
  Add1/1 -> Gain4/1
  Demux2/1 -> Terminator2/1
  Demux2/2 -> [a_MB]
  MB/1 -> Demux2/1
  Demux2/3 -> Terminator1/1
  Demux2/4 -> [h_MB]

== system detumbling1/External Torques/Solar radiation/Torque arm MB/creazione raggi vettore tra CM MB e centro facce illuminate della faccia che ha come normale l'asse j/If Action Subsystem3 ==
  Areas_vect : Inport
  MB : Inport  Port=2
  Action Port : ActionPort  ActionPortLabel=if(u1<0 & u2<0)
  Add : Sum  Inputs=+|-
  Add1 : Sum  Inputs=+|-
  Add2 : Sum
  Demux : Demux  Outputs=3
  Demux2 : Demux
  Divide : Product  Inputs=*/
  Divide1 : Product  Inputs=*/
  Gain{,1..3} (4 alike) : Gain  Gain=1/2
  Gain4 : Gain  Gain=-1
  Gain5 : Gain  Gain=-1
  Ground : Ground
  Ground1 : Ground
  Mux : Mux  Inputs=3
  Mux1 : Mux  Inputs=3
  Reshape : Reshape  OutputDimensionality=Column vector (2-D)
  Reshape2 : Reshape  OutputDimensionality=Column vector (2-D)
  Reshape3 : Reshape  OutputDimensionality=Column vector (2-D)
  Terminator{1..2,8..9} (4 alike) : Terminator
  r_cface_cluce_x_neg_z_neg : Outport
  wires:
  Add1/1 -> Gain4/1
  Gain4/1 -> Mux1/1
  Demux/3 -> Terminator8/1
  Demux/1 -> Terminator9/1
  Add2/1 -> r_cface_cluce_x_neg_z_neg/1
  Reshape3/1 -> Add2/2
  Reshape2/1 -> Add2/1
  [a_MB] -> Gain2/1
  Divide1/1 -> Gain3/1
  Gain2/1 -> Add1/1
  Gain3/1 -> Add1/2
  Ground/1 -> Mux1/3, Mux1/2
  Mux1/1 -> Reshape3/1  "raggio vettore che collega il centro geom della faccia con il centro geom della faccia illuminata dal sole lungo -i"
  [h_MB] -> Divide1/2
  Reshape/1 -> Demux/1
  Ground1/1 -> Mux/1, Mux/2
  Areas_vect/1 -> Reshape/1
  [a_MB] -> Divide/2
  Gain/1 -> Add/1
  [h_MB] -> Gain/1
  Demux/2 -> Divide/1, Divide1/1
  Gain1/1 -> Add/2
  Mux/1 -> Reshape2/1  "raggio vettore che collega il centro geom della faccia con il centro geom della faccia illuminata dal sole lungo -k"
  Divide/1 -> Gain1/1
  Add/1 -> Gain5/1
  Gain5/1 -> Mux/3
  Demux2/1 -> Terminator2/1
  Demux2/2 -> [a_MB]
  MB/1 -> Demux2/1
  Demux2/3 -> Terminator1/1
  Demux2/4 -> [h_MB]

== system detumbling1/External Torques/Solar radiation/Torque arm MB/creazione raggi vettore tra CM MB e centro facce illuminate della faccia che ha come normale l'asse j/If Action Subsystem4 ==
  Action Port : ActionPort  ActionPortLabel=else
  Constant : Constant  Value=[0;0;0]
  Out1 : Outport
  wires:
  Constant/1 -> Out1/1

== system detumbling1/External Torques/Solar radiation/Torque arm MB/creazione raggi vettore tra CM MB e centro facce illuminate della faccia che ha come normale l'asse j/If Action Subsystem5 ==
  Action Port : ActionPort  ActionPortLabel=else
  Constant : Constant  Value=[0;0;0]
  Out1 : Outport
  wires:
  Constant/1 -> Out1/1

== system detumbling1/External Torques/Solar radiation/Torque arm MB/creazione raggi vettore tra CM MB e centro facce illuminate della faccia che ha come normale l'asse j/If Action Subsystem6 ==
  Action Port : ActionPort  ActionPortLabel=else
  Constant : Constant  Value=[0;0;0]
  Out1 : Outport
  wires:
  Constant/1 -> Out1/1

== system detumbling1/External Torques/Solar radiation/Torque arm MB/creazione raggi vettore tra CM MB e centro facce illuminate della faccia che ha come normale l'asse j/If Action Subsystem7 ==
  Action Port : ActionPort  ActionPortLabel=else
  Constant : Constant  Value=[0;0;0]
  Out1 : Outport
  wires:
  Constant/1 -> Out1/1

== system detumbling1/External Torques/Solar radiation/Torque arm MB/creazione raggi vettore tra CM MB e centro facce illuminate della faccia che ha come normale l'asse j/creating distance between cm MB and centro geom lato1 ==
  MB : Inport
  pointer : Inport  Port=2
  Demux : Demux
  Ground : Ground
  Mux : Mux  Inputs=3
  Product : Product
  Reshape : Reshape  OutputDimensionality=Column vector (2-D)
  Terminator : Terminator
  Terminator1 : Terminator
  Terminator2 : Terminator
  Out1 : Outport
  wires:
  Reshape/1 -> Out1/1
  Mux/1 -> Reshape/1
  MB/1 -> Demux/1
  Demux/1 -> Terminator/1
  Demux/2 -> Terminator1/1
  Demux/3 -> Terminator2/1
  Ground/1 -> Mux/2, Mux/1
  Demux/4 -> Product/1
  pointer/1 -> Product/2
  Product/1 -> Mux/3

== system detumbling1/External Torques/Solar radiation/Torque arm MB/creazione raggi vettore tra CM MB e centro facce illuminate della faccia che ha come normale l'asse k/If Action Subsystem ==
  Areas_vect : Inport
  MB : Inport  Port=2
  Action Port : ActionPort  ActionPortLabel=if(u1>0 & u2>0)
  Add : Sum  Inputs=+|-
  Add1 : Sum  Inputs=+|-
  Add2 : Sum
  Demux : Demux  Outputs=3
  Demux1 : Demux  Outputs=3
  Demux2 : Demux
  Divide : Product  Inputs=*/
  Divide1 : Product  Inputs=*/
  Gain{,1..3} (4 alike) : Gain  Gain=1/2
  Ground : Ground
  Ground1 : Ground
  Mux : Mux  Inputs=3
  Mux1 : Mux  Inputs=3
  Reshape{,1..3} (4 alike) : Reshape  OutputDimensionality=Column vector (2-D)
  Terminator{,1..3,8..9} (6 alike) : Terminator
  r_cface_cluce_xy_pos : Outport
  wires:
  Add/1 -> Mux/2
  Divide/1 -> Gain1/1
  Mux/1 -> Reshape2/1  "raggio vettore che collega il centro geom della faccia con il centro geom della faccia illuminata dal sole lungo j"
  Gain1/1 -> Add/2
  Demux/3 -> Divide/1
  [b_MB] -> Gain/1
  Gain/1 -> Add/1
  [a_MB] -> Divide/2
  Areas_vect/1 -> Reshape/1, Reshape1/1
  Ground1/1 -> Mux/1, Mux/3
  Reshape/1 -> Demux/1
  Add1/1 -> Mux1/1
  [b_MB] -> Divide1/2
  Mux1/1 -> Reshape3/1  "raggio vettore che collega il centro geom della faccia con il centro geom della faccia illuminata dal sole lungo x"
  Ground/1 -> Mux1/2, Mux1/3
  Demux1/3 -> Divide1/1
  Gain3/1 -> Add1/2
  Gain2/1 -> Add1/1
  Reshape1/1 -> Demux1/1
  Divide1/1 -> Gain3/1
  [a_MB] -> Gain2/1
  Reshape2/1 -> Add2/1
  Reshape3/1 -> Add2/2
  Add2/1 -> r_cface_cluce_xy_pos/1
  Demux1/1 -> Terminator/1
  Demux1/2 -> Terminator1/1
  Demux/1 -> Terminator9/1
  Demux/2 -> Terminator8/1
  MB/1 -> Demux2/1
  Demux2/1 -> Terminator2/1
  Demux2/2 -> [a_MB]
  Demux2/3 -> [b_MB]
  Demux2/4 -> Terminator3/1

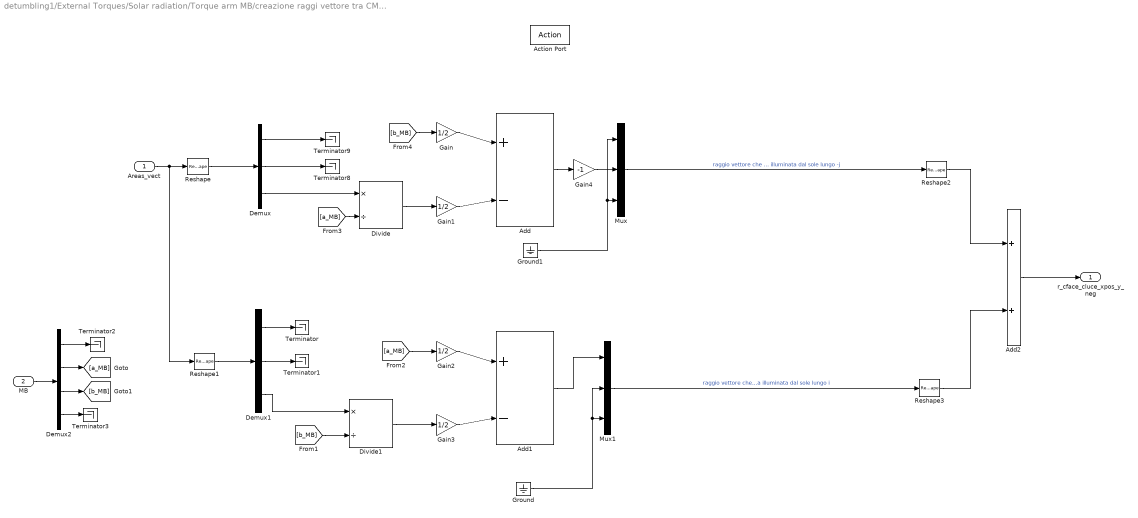
== system detumbling1/External Torques/Solar radiation/Torque arm MB/creazione raggi vettore tra CM MB e centro facce illuminate della faccia che ha come normale l'asse k/If Action Subsystem1 ==
  Areas_vect : Inport
  MB : Inport  Port=2
  Action Port : ActionPort  ActionPortLabel=if(u1>0 & u2<0)
  Add : Sum  Inputs=+|-
  Add1 : Sum  Inputs=+|-
  Add2 : Sum
  Demux : Demux  Outputs=3
  Demux1 : Demux  Outputs=3
  Demux2 : Demux
  Divide : Product  Inputs=*/
  Divide1 : Product  Inputs=*/
  Gain{,1..3} (4 alike) : Gain  Gain=1/2
  Gain4 : Gain  Gain=-1
  Ground : Ground
  Ground1 : Ground
  Mux : Mux  Inputs=3
  Mux1 : Mux  Inputs=3
  Reshape{,1..3} (4 alike) : Reshape  OutputDimensionality=Column vector (2-D)
  Terminator{,1..3,8..9} (6 alike) : Terminator
  r_cface_cluce_xpos_y_neg : Outport
  wires:
  Add/1 -> Gain4/1
  Divide/1 -> Gain1/1
  Mux/1 -> Reshape2/1  "raggio vettore che collega il centro geom della faccia con il centro geom della faccia illuminata dal sole lungo -j"
  Gain1/1 -> Add/2
  Demux/3 -> Divide/1
  Gain/1 -> Add/1
  Areas_vect/1 -> Reshape/1, Reshape1/1
  Ground1/1 -> Mux/1, Mux/3
  Reshape/1 -> Demux/1
  Mux1/1 -> Reshape3/1  "raggio vettore che collega il centro geom della faccia con il centro geom della faccia illuminata dal sole lungo i"
  Ground/1 -> Mux1/2, Mux1/3
  Demux1/3 -> Divide1/1
  Gain3/1 -> Add1/2
  Gain2/1 -> Add1/1
  Reshape1/1 -> Demux1/1
  Divide1/1 -> Gain3/1
  Reshape2/1 -> Add2/1
  Reshape3/1 -> Add2/2
  Add2/1 -> r_cface_cluce_xpos_y_neg/1
  Demux1/1 -> Terminator/1
  Demux1/2 -> Terminator1/1
  Demux/1 -> Terminator9/1
  Demux/2 -> Terminator8/1
  Gain4/1 -> Mux/2
  [a_MB] -> Divide/2
  [b_MB] -> Gain/1
  Add1/1 -> Mux1/1
  [b_MB] -> Divide1/2
  [a_MB] -> Gain2/1
  Demux2/1 -> Terminator2/1
  Demux2/2 -> [a_MB]
  MB/1 -> Demux2/1
  Demux2/3 -> [b_MB]
  Demux2/4 -> Terminator3/1

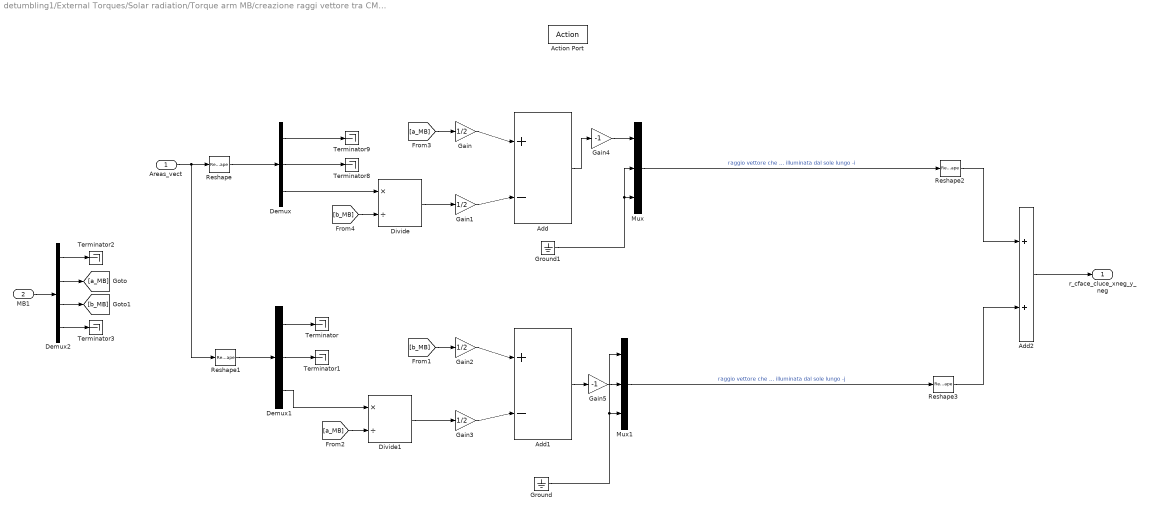
== system detumbling1/External Torques/Solar radiation/Torque arm MB/creazione raggi vettore tra CM MB e centro facce illuminate della faccia che ha come normale l'asse k/If Action Subsystem2 ==
  Areas_vect : Inport
  MB1 : Inport  Port=2
  Action Port : ActionPort  ActionPortLabel=if(u1<0 & u2<0)
  Add : Sum  Inputs=+|-
  Add1 : Sum  Inputs=+|-
  Add2 : Sum
  Demux : Demux  Outputs=3
  Demux1 : Demux  Outputs=3
  Demux2 : Demux
  Divide : Product  Inputs=*/
  Divide1 : Product  Inputs=*/
  Gain{,1..3} (4 alike) : Gain  Gain=1/2
  Gain4 : Gain  Gain=-1
  Gain5 : Gain  Gain=-1
  Ground : Ground
  Ground1 : Ground
  Mux : Mux  Inputs=3
  Mux1 : Mux  Inputs=3
  Reshape{,1..3} (4 alike) : Reshape  OutputDimensionality=Column vector (2-D)
  Terminator{,1..3,8..9} (6 alike) : Terminator
  r_cface_cluce_xneg_y_neg : Outport
  wires:
  [a_MB] -> Divide1/2
  [b_MB] -> Gain2/1
  Add1/1 -> Gain5/1
  Gain4/1 -> Mux/1
  Add/1 -> Gain4/1
  [a_MB] -> Gain/1
  [b_MB] -> Divide/2
  Divide/1 -> Gain1/1
  Mux/1 -> Reshape2/1  "raggio vettore che collega il centro geom della faccia con il centro geom della faccia illuminata dal sole lungo -i"
  Gain1/1 -> Add/2
  Demux/3 -> Divide/1
  Gain/1 -> Add/1
  Areas_vect/1 -> Reshape/1, Reshape1/1
  Ground1/1 -> Mux/3, Mux/2
  Reshape/1 -> Demux/1
  Mux1/1 -> Reshape3/1  "raggio vettore che collega il centro geom della faccia con il centro geom della faccia illuminata dal sole lungo -j"
  Ground/1 -> Mux1/3, Mux1/1
  Demux1/3 -> Divide1/1
  Gain3/1 -> Add1/2
  Gain2/1 -> Add1/1
  Reshape1/1 -> Demux1/1
  Divide1/1 -> Gain3/1
  Reshape2/1 -> Add2/1
  Reshape3/1 -> Add2/2
  Add2/1 -> r_cface_cluce_xneg_y_neg/1
  Demux1/1 -> Terminator/1
  Demux1/2 -> Terminator1/1
  Demux/1 -> Terminator9/1
  Demux/2 -> Terminator8/1
  Gain5/1 -> Mux1/2
  Demux2/1 -> Terminator2/1
  Demux2/2 -> [a_MB]
  MB1/1 -> Demux2/1
  Demux2/3 -> [b_MB]
  Demux2/4 -> Terminator3/1

== system detumbling1/External Torques/Solar radiation/Torque arm MB/creazione raggi vettore tra CM MB e centro facce illuminate della faccia che ha come normale l'asse k/If Action Subsystem3 ==
  Action Port : ActionPort  ActionPortLabel=else
  Constant : Constant  Value=[0;0;0]
  Out1 : Outport
  wires:
  Constant/1 -> Out1/1
